simulink model "Arduino_PID_Interface2015b"  (R2015b)
settings: Solver=VariableStepAuto  SolverMode=SingleTasking  StartTime=0.0  StopTime=inf  RelTol=1e-3
undefined symbols (not defined in the file or in its folder): LF, serial
libraries: instrumentlib x3
settings Model: Creator=VM  LastModifiedBy=rap.kuttruf.17
settings DataIOCC: LimitDataPoints=off  ReturnWorkspaceOutputs=on
settings DebuggingCC: AllowSymbolicDim=on  SFUnexpectedBacktrackingDiag=error  SFNoUnconditionalDefaultTransitionDiag=error
settings ModelReferenceCC: PropagateSignalLabelsOutOfModel=on
settings SFSimCC: SimUseLocalCustomCode=on
settings RTWCC: RTWUseLocalCustomCode=on
settings GRTTargetCC: TargetLangStandard=C99 (ISO)
settings ConfigComp: CovMetricSettings=dwe  CovHtmlReporting=off  CovSaveCumulativeToWorkspaceVar=off  CovSaveSingleToWorkspaceVar=off  CovModelRefEnable=Off  CovExternalEMLEnable=on

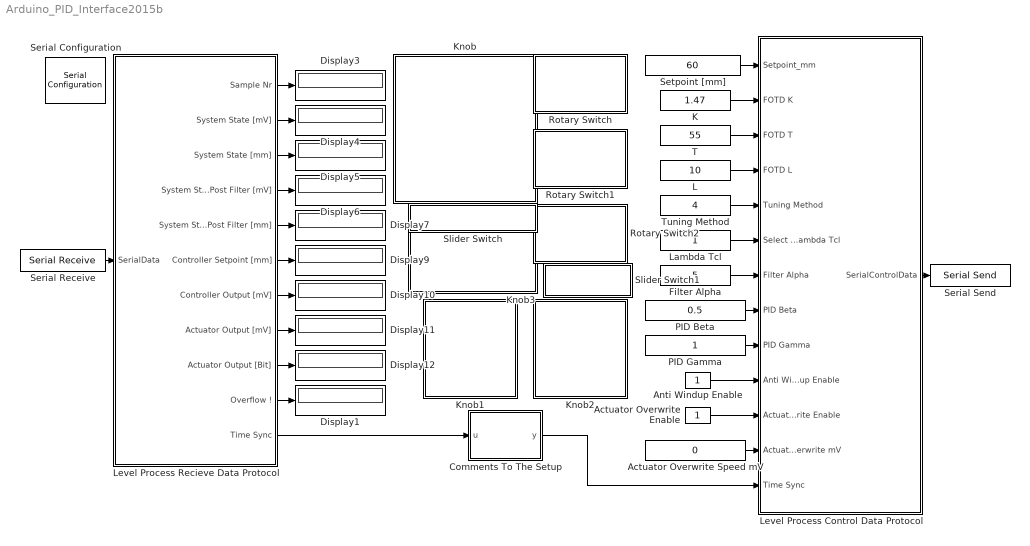
== system Arduino_PID_Interface2015b ==
  Actuator Overwrite Enable : Constant  OutDataTypeStr=uint8
  Actuator Overwrite Speed mV : Constant  Value=0  OutDataTypeStr=double
  Anti Windup Enable : Constant  OutDataTypeStr=uint8
  Comments To The Setup : MATLAB Function  TreatAsAtomicUnit=on
  Display{1,3..7,9..12} (10 alike) : Display
  Filter Alpha : Constant  Value=5
  K : Constant  Value=1.47
  Knob : Subsystem  DialogController=hmiCreateDDGDialog  IsWebBlock=on  mask(MWDashboardBlock){webBlockId=6f032d83-7110-46a9-9e70-2962474ee83c, webBlockType=continuousknob, ShowInLibBrowser=on, ShowInitialText=on, HMISrcModelName=Arduino_PID_Interface2015b}
      mask prompts: webBlockId "WebBlock Id"; webBlockType "WebBlock Type"; HMISrcModelName "Source Model"
      mask help: Set a value to tune parameters or variables.
      mask Help: helpview([docroot '/mapfiles/simulink.map'], 'hmi_knob')
      mask Display:
      | if strcmp(get_param(bdroot(gcb),'BlockDiagramType'),'library')
      |  image([(matlabroot) '/toolbox/simulink/hmi/icons/ContinuousKnob.png'])
      | end
  Knob1 : Subsystem  DialogController=hmiCreateDDGDialog  IsWebBlock=on  mask(MWDashboardBlock){webBlockId=2d92fb6d-6817-4e61-8a75-49afcc5cee09, webBlockType=continuousknob, ShowInLibBrowser=on, ShowInitialText=on, HMISrcModelName=Arduino_PID_Interface2015b}
      mask prompts: webBlockId "WebBlock Id"; webBlockType "WebBlock Type"; HMISrcModelName "Source Model"
      mask help: Set a value to tune parameters or variables.
      mask Help: helpview([docroot '/mapfiles/simulink.map'], 'hmi_knob')
      mask Display:
      | if strcmp(get_param(bdroot(gcb),'BlockDiagramType'),'library')
      |  image([(matlabroot) '/toolbox/simulink/hmi/icons/ContinuousKnob.png'])
      | end
  Knob2 : Subsystem  DialogController=hmiCreateDDGDialog  IsWebBlock=on  mask(MWDashboardBlock){webBlockId=b3bbeefb-f65b-4d0a-99f2-2d47ca17d880, webBlockType=continuousknob, ShowInLibBrowser=on, ShowInitialText=on, HMISrcModelName=Arduino_PID_Interface2015b}
      mask prompts: webBlockId "WebBlock Id"; webBlockType "WebBlock Type"; HMISrcModelName "Source Model"
      mask help: Set a value to tune parameters or variables.
      mask Help: helpview([docroot '/mapfiles/simulink.map'], 'hmi_knob')
      mask Display:
      | if strcmp(get_param(bdroot(gcb),'BlockDiagramType'),'library')
      |  image([(matlabroot) '/toolbox/simulink/hmi/icons/ContinuousKnob.png'])
      | end
  Knob3 : Subsystem  DialogController=hmiCreateDDGDialog  IsWebBlock=on  mask(MWDashboardBlock){webBlockId=3082382d-e086-4832-b15c-b96756403168, webBlockType=continuousknob, ShowInLibBrowser=on, ShowInitialText=on, HMISrcModelName=Arduino_PID_Interface2015b}
      mask prompts: webBlockId "WebBlock Id"; webBlockType "WebBlock Type"; HMISrcModelName "Source Model"
      mask help: Set a value to tune parameters or variables.
      mask Help: helpview([docroot '/mapfiles/simulink.map'], 'hmi_knob')
      mask Display:
      | if strcmp(get_param(bdroot(gcb),'BlockDiagramType'),'library')
      |  image([(matlabroot) '/toolbox/simulink/hmi/icons/ContinuousKnob.png'])
      | end
  L : Constant  Value=10
  Lambda Tcl : Constant
  Level Process Control Data Protocol : Subsystem
  Level Process Recieve Data Protocol : Subsystem
  PID Beta : Constant  Value=0.5
  PID Gamma : Constant
  Rotary Switch : Subsystem  DialogController=hmiCreateDDGDialog  IsWebBlock=on  mask(MWDashboardBlock){webBlockId=54f21b2c-51f9-4bca-8c45-8dfda734ad71, webBlockType=discreteknob, ShowInLibBrowser=on, ShowInitialText=on, HMISrcModelName=Arduino_PID_Interface2015b}
      mask prompts: webBlockId "WebBlock Id"; webBlockType "WebBlock Type"; HMISrcModelName "Source Model"
      mask help: Set value to tune parameters or variables.
      mask Help: helpview([docroot '/mapfiles/simulink.map'], 'hmi_rotary_switch')
      mask Display:
      | if strcmp(get_param(bdroot(gcb),'BlockDiagramType'),'library')
      |  image([(matlabroot) '/toolbox/simulink/hmi/icons/DiscreteKnob.png'])
      | end
  Rotary Switch1 : Subsystem  DialogController=hmiCreateDDGDialog  IsWebBlock=on  mask(MWDashboardBlock){webBlockId=c8a1b7f9-55eb-45f6-8afb-eb5ab7323296, webBlockType=discreteknob, ShowInLibBrowser=on, ShowInitialText=on, HMISrcModelName=Arduino_PID_Interface2015b}
      mask prompts: webBlockId "WebBlock Id"; webBlockType "WebBlock Type"; HMISrcModelName "Source Model"
      mask help: Set value to tune parameters or variables.
      mask Help: helpview([docroot '/mapfiles/simulink.map'], 'hmi_rotary_switch')
      mask Display:
      | if strcmp(get_param(bdroot(gcb),'BlockDiagramType'),'library')
      |  image([(matlabroot) '/toolbox/simulink/hmi/icons/DiscreteKnob.png'])
      | end
  Rotary Switch2 : Subsystem  DialogController=hmiCreateDDGDialog  IsWebBlock=on  mask(MWDashboardBlock){webBlockId=0e63494c-69fc-4820-84ef-30df04359523, webBlockType=discreteknob, ShowInLibBrowser=on, ShowInitialText=on, HMISrcModelName=Arduino_PID_Interface2015b}
      mask prompts: webBlockId "WebBlock Id"; webBlockType "WebBlock Type"; HMISrcModelName "Source Model"
      mask help: Set value to tune parameters or variables.
      mask Help: helpview([docroot '/mapfiles/simulink.map'], 'hmi_rotary_switch')
      mask Display:
      | if strcmp(get_param(bdroot(gcb),'BlockDiagramType'),'library')
      |  image([(matlabroot) '/toolbox/simulink/hmi/icons/DiscreteKnob.png'])
      | end
  Serial Configuration : instrumentlib/Serial Configuration  Priority=-200000  ComPortMenu=<Please select a port...>  ComPort=COM5  ObjConstructor=serial('COM5');  BaudRate=115200  DataBits=8  Parity=none  StopBits=1  FlowControl=none  Timeout=10  ByteOrder=LittleEndian
  Serial Receive : instrumentlib/Serial Receive  ComPortMenu=<Please select a port...>  ComPort=COM5  ObjConstructor=serial('COM5');  Header=<D>  Terminator=LF ('\n')  DataSize="[1  32]"  DataType=uint8  EnableBlockingMode=on  ActionDataUnavailable=Output last received value  CustomValue=0  SampleTime=0.001
  Serial Send : instrumentlib/Serial Send  ComPortMenu=<Please select a port...>  ComPort=COM5  ObjConstructor=serial('COM5');  Header=<C>  Terminator=LF ('\n')  EnableBlockingMode=on
  Setpoint [mm] : Constant  Value=60  OutDataTypeStr=uint16
  Slider Switch : Subsystem  DialogController=hmiCreateDDGDialog  IsWebBlock=on  mask(MWDashboardBlock){webBlockId=4b07397e-e0fe-4bf8-b10b-d486fcba6875, webBlockType=sliderswitch, ShowInLibBrowser=on, ShowInitialText=on, HMISrcModelName=Arduino_PID_Interface2015b}
      mask prompts: webBlockId "WebBlock Id"; webBlockType "WebBlock Type"; HMISrcModelName "Source Model"
      mask help: Set on/off value to tune parameters or variables.
      mask Help: helpview([docroot '/mapfiles/simulink.map'], 'hmi_switch')
      mask Display:
      | if strcmp(get_param(bdroot(gcb),'BlockDiagramType'),'library')
      |  image([(matlabroot) '/toolbox/simulink/hmi/icons/SliderSwitch.png'])
      | end
  Slider Switch1 : Subsystem  DialogController=hmiCreateDDGDialog  IsWebBlock=on  mask(MWDashboardBlock){webBlockId=f5a7a057-55eb-455d-becd-9f4f82eab9b0, webBlockType=sliderswitch, ShowInLibBrowser=on, ShowInitialText=on, HMISrcModelName=Arduino_PID_Interface2015b}
      mask prompts: webBlockId "WebBlock Id"; webBlockType "WebBlock Type"; HMISrcModelName "Source Model"
      mask help: Set on/off value to tune parameters or variables.
      mask Help: helpview([docroot '/mapfiles/simulink.map'], 'hmi_switch')
      mask Display:
      | if strcmp(get_param(bdroot(gcb),'BlockDiagramType'),'library')
      |  image([(matlabroot) '/toolbox/simulink/hmi/icons/SliderSwitch.png'])
      | end
  T : Constant  Value=55
  Tuning Method : Constant  Value=4
  wires:
  Serial Receive/1 -> Level Process Recieve Data Protocol/1(SerialData)
  Setpoint [mm]/1 -> Level Process Control Data Protocol/1(Setpoint_mm)
  Level Process Recieve Data Protocol/1(Sample Nr) -> Display3/1
  Level Process Recieve Data Protocol/2(System State [mV]) -> Display4/1
  Level Process Recieve Data Protocol/3(System State [mm]) -> Display5/1
  Level Process Recieve Data Protocol/4(System State Post Filter [mV]) -> Display6/1
  Level Process Recieve Data Protocol/5(System State Post Filter [mm]) -> Display7/1
  Level Process Recieve Data Protocol/6(Controller Setpoint [mm]) -> Display9/1
  Level Process Recieve Data Protocol/7(Controller Output [mV]) -> Display10/1
  Level Process Recieve Data Protocol/8(Actuator Output [mV]) -> Display11/1
  Level Process Recieve Data Protocol/9(Actuator Output [Bit]) -> Display12/1
  Tuning Method/1 -> Level Process Control Data Protocol/5(Tuning Method)
  Filter Alpha/1 -> Level Process Control Data Protocol/7(Filter Alpha)
  Level Process Control Data Protocol/1(SerialControlData) -> Serial Send/1
  K/1 -> Level Process Control Data Protocol/2(FOTD K)
  PID Beta/1 -> Level Process Control Data Protocol/8(PID Beta)
  PID Gamma/1 -> Level Process Control Data Protocol/9(PID Gamma)
  T/1 -> Level Process Control Data Protocol/3(FOTD T)
  L/1 -> Level Process Control Data Protocol/4(FOTD L)
  Lambda Tcl/1 -> Level Process Control Data Protocol/6(Select Lambda Tcl)
  Level Process Recieve Data Protocol/11(Time Sync) -> Comments To The Setup/1(u)
  Comments To The Setup/1(y) -> Level Process Control Data Protocol/13(Time Sync)
  Level Process Recieve Data Protocol/10(Overflow !) -> Display1/1
  Actuator Overwrite Speed mV/1 -> Level Process Control Data Protocol/12(Actuator Speed Overwrite mV)
  Actuator Overwrite Enable/1 -> Level Process Control Data Protocol/11(Actuator Overwrite Enable)
  Anti Windup Enable/1 -> Level Process Control Data Protocol/10(Anti Windup Enable)

== system Arduino_PID_Interface2015b/Knob ==

== system Arduino_PID_Interface2015b/Knob1 ==

== system Arduino_PID_Interface2015b/Knob2 ==

== system Arduino_PID_Interface2015b/Knob3 ==

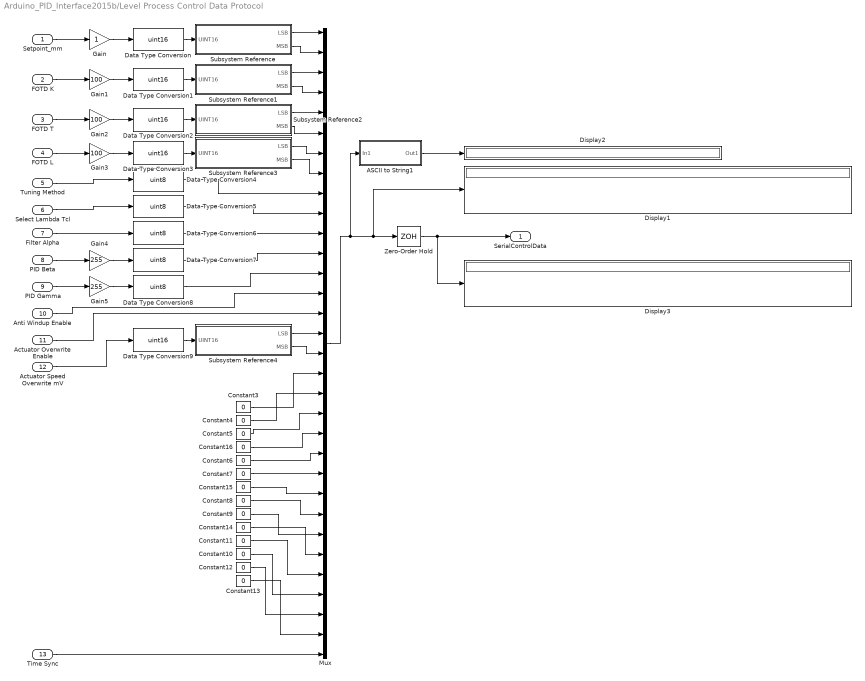
== system Arduino_PID_Interface2015b/Level Process Control Data Protocol ==
  Setpoint_mm : Inport
  FOTD K : Inport  Port=2
  FOTD T : Inport  Port=3
  FOTD L : Inport  Port=4
  Tuning Method : Inport  Port=5
  Select Lambda Tcl : Inport  Port=6
  Filter Alpha : Inport  Port=7
  PID Beta : Inport  Port=8
  PID Gamma : Inport  Port=9
  Anti Windup Enable : Inport  Port=10
  Actuator Overwrite Enable : Inport  Port=11
  Actuator Speed Overwrite mV : Inport  Port=12
  Time Sync : Inport  Port=13
  ASCII to String1 : Subsystem  Description=Replaced Block  mask(Replaced Block){}
      mask help: This block has been replaced with an empty subsystem because it used functionality that is unavailable in Simulink R2015b.
      mask Display: fprintf('Replaced: %s\n','ASCIIToString')
  Constant{3..16} (14 alike) : Constant  Value=0  OutDataTypeStr=uint8
  Data Type Conversion{,1..3,9} (5 alike) : DataTypeConversion  OutDataTypeStr=uint16
  Data Type Conversion{4..8} (5 alike) : DataTypeConversion  OutDataTypeStr=uint8
  Display1 : Display
      settings: Decimation=32
  Display2 : Display
  Display3 : Display
      settings: Decimation=32
  Gain : Gain
  Gain1 : Gain  Gain=100
  Gain2 : Gain  Gain=100
  Gain3 : Gain  Gain=100
  Gain4 : Gain  Gain=255
  Gain5 : Gain  Gain=255
  Mux : Mux  Inputs=32
  Subsystem Reference : Subsystem
  Subsystem Reference1 : Subsystem
  Subsystem Reference2 : Subsystem
  Subsystem Reference3 : Subsystem
  Subsystem Reference4 : Subsystem
  Zero-Order Hold : ZeroOrderHold  SampleTime=0.005
  SerialControlData : Outport
  wires:
  Subsystem Reference/1(LSB) -> Mux/1
  Subsystem Reference/2(MSB) -> Mux/2
  Data Type Conversion/1 -> Subsystem Reference/1(UINT16)
  Gain/1 -> Data Type Conversion/1
  Setpoint_mm/1 -> Gain/1
  Gain1/1 -> Data Type Conversion1/1
  Data Type Conversion1/1 -> Subsystem Reference1/1(UINT16)
  Subsystem Reference1/1(LSB) -> Mux/3
  Subsystem Reference1/2(MSB) -> Mux/4
  Gain2/1 -> Data Type Conversion2/1
  Data Type Conversion2/1 -> Subsystem Reference2/1(UINT16)
  Subsystem Reference2/1(LSB) -> Mux/5
  Subsystem Reference2/2(MSB) -> Mux/6
  Gain3/1 -> Data Type Conversion3/1
  Data Type Conversion3/1 -> Subsystem Reference3/1(UINT16)
  Subsystem Reference3/1(LSB) -> Mux/7
  Subsystem Reference3/2(MSB) -> Mux/8
  FOTD K/1 -> Gain1/1
  FOTD T/1 -> Gain2/1
  FOTD L/1 -> Gain3/1
  Tuning Method/1 -> Data Type Conversion4/1
  Data Type Conversion4/1 -> Mux/9
  Select Lambda Tcl/1 -> Data Type Conversion5/1
  Filter Alpha/1 -> Data Type Conversion6/1
  Data Type Conversion5/1 -> Mux/10
  Data Type Conversion6/1 -> Mux/11
  Data Type Conversion7/1 -> Mux/12
  Data Type Conversion8/1 -> Mux/13
  ASCII to String1/1(Out1) -> Display2/1
  Mux/1 -> ASCII to String1/1(In1), Zero-Order Hold/1, Display1/1
  PID Beta/1 -> Gain4/1
  Gain4/1 -> Data Type Conversion7/1
  PID Gamma/1 -> Gain5/1
  Gain5/1 -> Data Type Conversion8/1
  Time Sync/1 -> Mux/32
  Constant3/1 -> Mux/18
  Constant4/1 -> Mux/19
  Constant5/1 -> Mux/20
  Constant6/1 -> Mux/22
  Constant7/1 -> Mux/23
  Constant8/1 -> Mux/25
  Constant9/1 -> Mux/26
  Constant10/1 -> Mux/29
  Constant11/1 -> Mux/28
  Constant12/1 -> Mux/30
  Constant13/1 -> Mux/31
  Constant15/1 -> Mux/24
  Constant16/1 -> Mux/21
  Constant14/1 -> Mux/27
  Data Type Conversion9/1 -> Subsystem Reference4/1(UINT16)
  Actuator Speed Overwrite mV/1 -> Data Type Conversion9/1
  Zero-Order Hold/1 -> Display3/1, SerialControlData/1
  Subsystem Reference4/1(LSB) -> Mux/16
  Subsystem Reference4/2(MSB) -> Mux/17
  Actuator Overwrite Enable/1 -> Mux/15
  Anti Windup Enable/1 -> Mux/14

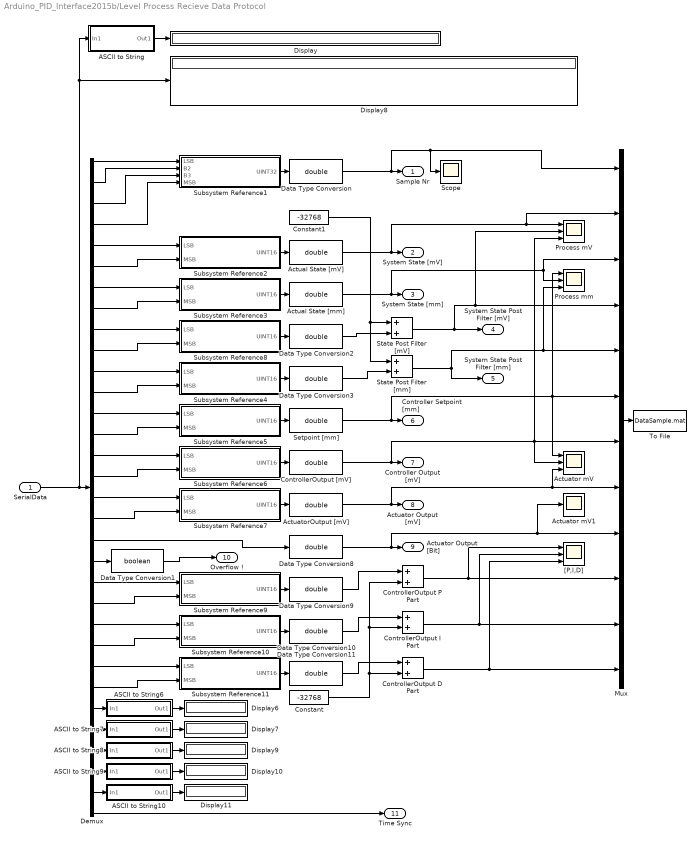
== system Arduino_PID_Interface2015b/Level Process Recieve Data Protocol ==
  SerialData : Inport
  " Actual State [mV]" : DataTypeConversion  OutDataTypeStr=double
  " Actual State [mm]" : DataTypeConversion  OutDataTypeStr=double
  ASCII to String : Subsystem  Description=Replaced Block  mask(Replaced Block){}
      mask help: This block has been replaced with an empty subsystem because it used functionality that is unavailable in Simulink R2015b.
      mask Display: fprintf('Replaced: %s\n','ASCIIToString')
  ASCII to String10 : Subsystem  Description=Replaced Block  mask(Replaced Block){}
      mask help: This block has been replaced with an empty subsystem because it used functionality that is unavailable in Simulink R2015b.
      mask Display: fprintf('Replaced: %s\n','ASCIIToString')
  ASCII to String6 : Subsystem  Description=Replaced Block  mask(Replaced Block){}
      mask help: This block has been replaced with an empty subsystem because it used functionality that is unavailable in Simulink R2015b.
      mask Display: fprintf('Replaced: %s\n','ASCIIToString')
  ASCII to String7 : Subsystem  Description=Replaced Block  mask(Replaced Block){}
      mask help: This block has been replaced with an empty subsystem because it used functionality that is unavailable in Simulink R2015b.
      mask Display: fprintf('Replaced: %s\n','ASCIIToString')
  ASCII to String8 : Subsystem  Description=Replaced Block  mask(Replaced Block){}
      mask help: This block has been replaced with an empty subsystem because it used functionality that is unavailable in Simulink R2015b.
      mask Display: fprintf('Replaced: %s\n','ASCIIToString')
  ASCII to String9 : Subsystem  Description=Replaced Block  mask(Replaced Block){}
      mask help: This block has been replaced with an empty subsystem because it used functionality that is unavailable in Simulink R2015b.
      mask Display: fprintf('Replaced: %s\n','ASCIIToString')
  Actuator mV : Scope  NumInputPorts=3
  Actuator mV1 : Scope
  ActuatorOutput [mV] : DataTypeConversion  OutDataTypeStr=double
  Constant : Constant  Value=-32768
  Constant1 : Constant  Value=-32768
  ControllerOutput D Part : Sum
  ControllerOutput I Part : Sum
  ControllerOutput P Part : Sum
  ControllerOutput [mV] : DataTypeConversion  OutDataTypeStr=double
  Data Type Conversion{,2..3,8..11} (7 alike) : DataTypeConversion  OutDataTypeStr=double
  Data Type Conversion1 : DataTypeConversion  OutDataTypeStr=boolean
  Demux : Demux  Outputs=32
  Display{,6..11} (7 alike) : Display
      Display8 settings: Decimation=32
  Mux : Mux  Inputs=12
  Process mV : Scope  NumInputPorts=3
  Process mm : Scope  NumInputPorts=3
  Scope : Scope
  Setpoint [mm] : DataTypeConversion  OutDataTypeStr=double
  State Post Filter [mV] : Sum
  State Post Filter [mm] : Sum
  Subsystem Reference1 : Subsystem
  Subsystem Reference10 : Subsystem
  Subsystem Reference11 : Subsystem
  Subsystem Reference2 : Subsystem
  Subsystem Reference3 : Subsystem
  Subsystem Reference4 : Subsystem
  Subsystem Reference5 : Subsystem
  Subsystem Reference6 : Subsystem
  Subsystem Reference7 : Subsystem
  Subsystem Reference8 : Subsystem
  Subsystem Reference9 : Subsystem
  To File : ToFile  Filename=DataSample.mat  MatrixName=DataSample  SaveFormat=Timeseries
  "[P,I,D]" : Scope  NumInputPorts=3
  Sample Nr : Outport
  System State [mV] : Outport  Port=2
  System State [mm] : Outport  Port=3
  System State Post Filter [mV] : Outport  Port=4
  System State Post Filter [mm] : Outport  Port=5
  Controller Setpoint [mm] : Outport  Port=6
  Controller Output [mV] : Outport  Port=7
  Actuator Output [mV] : Outport  Port=8
  Actuator Output [Bit] : Outport  Port=9
  Overflow ! : Outport  Port=10  OutDataTypeStr=boolean
  Time Sync : Outport  Port=11
  wires:
  SerialData/1 -> ASCII to String/1(In1), Display8/1, Demux/1
  Demux/2 -> Subsystem Reference1/2(B2)
  Demux/1 -> Subsystem Reference1/1(LSB)
  Demux/3 -> Subsystem Reference1/3(B3)
  Demux/4 -> Subsystem Reference1/4(MSB)
  Demux/17 -> Subsystem Reference7/1(LSB)
  Demux/18 -> Subsystem Reference7/2(MSB)
  Subsystem Reference1/1(UINT32) -> Data Type Conversion/1
  Subsystem Reference7/1(UINT16) -> ActuatorOutput [mV]/1
  Demux/19 -> Data Type Conversion8/1
  Data Type Conversion/1 -> Scope/1, Mux/1, Sample Nr/1
  " Actual State [mV]"/1 -> Mux/2, Process mV/1, System State [mV]/1
  " Actual State [mm]"/1 -> Process mm/2, Mux/3, System State [mm]/1
  Setpoint [mm]/1 -> Process mm/1, Mux/6, Actuator mV/1, Controller Setpoint [mm]/1
  ControllerOutput [mV]/1 -> Actuator mV/2, Mux/7, Process mV/3, Controller Output [mV]/1
  ActuatorOutput [mV]/1 -> Actuator mV/3, Mux/8, Actuator Output [mV]/1
  Data Type Conversion8/1 -> Actuator mV1/1, Mux/9, Actuator Output [Bit]/1
  ASCII to String/1(Out1) -> Display/1
  Mux/1 -> To File/1
  Demux/32 -> Time Sync/1
  ASCII to String6/1(Out1) -> Display6/1
  Demux/27 -> ASCII to String6/1(In1)
  ASCII to String7/1(Out1) -> Display7/1
  Demux/28 -> ASCII to String7/1(In1)
  ASCII to String8/1(Out1) -> Display9/1
  Demux/29 -> ASCII to String8/1(In1)
  ASCII to String9/1(Out1) -> Display10/1
  Demux/30 -> ASCII to String9/1(In1)
  ASCII to String10/1(Out1) -> Display11/1
  Demux/31 -> ASCII to String10/1(In1)
  Subsystem Reference2/1(UINT16) -> " Actual State [mV]"/1
  Subsystem Reference3/1(UINT16) -> " Actual State [mm]"/1
  Subsystem Reference5/1(UINT16) -> Setpoint [mm]/1
  Subsystem Reference6/1(UINT16) -> ControllerOutput [mV]/1
  Demux/5 -> Subsystem Reference2/1(LSB)
  Demux/6 -> Subsystem Reference2/2(MSB)
  Demux/7 -> Subsystem Reference3/1(LSB)
  Demux/9 -> Subsystem Reference8/1(LSB)
  Demux/11 -> Subsystem Reference4/1(LSB)
  Demux/13 -> Subsystem Reference5/1(LSB)
  Demux/15 -> Subsystem Reference6/1(LSB)
  Demux/16 -> Subsystem Reference6/2(MSB)
  Demux/14 -> Subsystem Reference5/2(MSB)
  Demux/12 -> Subsystem Reference4/2(MSB)
  Demux/10 -> Subsystem Reference8/2(MSB)
  Demux/8 -> Subsystem Reference3/2(MSB)
  Demux/21 -> Subsystem Reference9/1(LSB)
  Demux/22 -> Subsystem Reference9/2(MSB)
  Demux/23 -> Subsystem Reference10/1(LSB)
  Demux/24 -> Subsystem Reference10/2(MSB)
  Demux/25 -> Subsystem Reference11/1(LSB)
  Demux/26 -> Subsystem Reference11/2(MSB)
  Subsystem Reference9/1(UINT16) -> Data Type Conversion9/1
  Subsystem Reference10/1(UINT16) -> Data Type Conversion10/1
  Subsystem Reference11/1(UINT16) -> Data Type Conversion11/1
  Data Type Conversion9/1 -> ControllerOutput P Part/1
  Data Type Conversion11/1 -> ControllerOutput D Part/1
  Data Type Conversion10/1 -> ControllerOutput I Part/1
  Constant/1 -> ControllerOutput D Part/2, ControllerOutput I Part/2, ControllerOutput P Part/2
  ControllerOutput P Part/1 -> "[P,I,D]"/1, Mux/10
  ControllerOutput I Part/1 -> "[P,I,D]"/2, Mux/11
  ControllerOutput D Part/1 -> Mux/12, "[P,I,D]"/3
  Data Type Conversion1/1 -> Overflow !/1
  Demux/20 -> Data Type Conversion1/1
  State Post Filter [mV]/1 -> System State Post Filter [mV]/1, Mux/4, Process mV/2
  Constant1/1 -> State Post Filter [mV]/1, State Post Filter [mm]/1
  Subsystem Reference8/1(UINT16) -> Data Type Conversion2/1
  Data Type Conversion2/1 -> State Post Filter [mV]/2
  Subsystem Reference4/1(UINT16) -> Data Type Conversion3/1
  Data Type Conversion3/1 -> State Post Filter [mm]/2
  State Post Filter [mm]/1 -> Mux/5, Process mm/3, System State Post Filter [mm]/1

== system Arduino_PID_Interface2015b/Rotary Switch ==

== system Arduino_PID_Interface2015b/Rotary Switch1 ==

== system Arduino_PID_Interface2015b/Rotary Switch2 ==

== system Arduino_PID_Interface2015b/Slider Switch ==

== system Arduino_PID_Interface2015b/Slider Switch1 ==

== system Arduino_PID_Interface2015b/Level Process Control Data Protocol/ASCII to String1 ==
  In1 : Inport
  Ground1 : Ground
  Terminator1 : Terminator
  Out1 : Outport
  wires:
  Ground1/1 -> Out1/1
  In1/1 -> Terminator1/1

== system Arduino_PID_Interface2015b/Level Process Control Data Protocol/Subsystem Reference ==
  UINT16 : Inport  OutDataTypeStr=uint16
  Data Type Conversion : DataTypeConversion  OutDataTypeStr=uint8
  Data Type Conversion1 : DataTypeConversion  OutDataTypeStr=uint8
  Data Type Conversion2 : DataTypeConversion  OutDataTypeStr=uint8  ConvertRealWorld=Stored Integer (SI)
  Display{,1..3} (4 alike) : Display
  Shift Arithmetic : ArithShift  BitShiftNumber=8  BitShiftDirection=Right
  LSB : Outport
  MSB : Outport  Port=2
  wires:
  Data Type Conversion2/1 -> Data Type Conversion/1, Display/1
  Data Type Conversion/1 -> LSB/1, Display2/1
  Data Type Conversion1/1 -> MSB/1, Display3/1
  Shift Arithmetic/1 -> Data Type Conversion1/1, Display1/1
  UINT16/1 -> Shift Arithmetic/1, Data Type Conversion2/1

== system Arduino_PID_Interface2015b/Level Process Control Data Protocol/Subsystem Reference1 ==
  UINT16 : Inport  OutDataTypeStr=uint16
  Data Type Conversion : DataTypeConversion  OutDataTypeStr=uint8
  Data Type Conversion1 : DataTypeConversion  OutDataTypeStr=uint8
  Data Type Conversion2 : DataTypeConversion  OutDataTypeStr=uint8  ConvertRealWorld=Stored Integer (SI)
  Display{,1..3} (4 alike) : Display
  Shift Arithmetic : ArithShift  BitShiftNumber=8  BitShiftDirection=Right
  LSB : Outport
  MSB : Outport  Port=2
  wires:
  Data Type Conversion2/1 -> Data Type Conversion/1, Display/1
  Data Type Conversion/1 -> LSB/1, Display2/1
  Data Type Conversion1/1 -> MSB/1, Display3/1
  Shift Arithmetic/1 -> Data Type Conversion1/1, Display1/1
  UINT16/1 -> Shift Arithmetic/1, Data Type Conversion2/1

== system Arduino_PID_Interface2015b/Level Process Control Data Protocol/Subsystem Reference2 ==
  UINT16 : Inport  OutDataTypeStr=uint16
  Data Type Conversion : DataTypeConversion  OutDataTypeStr=uint8
  Data Type Conversion1 : DataTypeConversion  OutDataTypeStr=uint8
  Data Type Conversion2 : DataTypeConversion  OutDataTypeStr=uint8  ConvertRealWorld=Stored Integer (SI)
  Display{,1..3} (4 alike) : Display
  Shift Arithmetic : ArithShift  BitShiftNumber=8  BitShiftDirection=Right
  LSB : Outport
  MSB : Outport  Port=2
  wires:
  Data Type Conversion2/1 -> Data Type Conversion/1, Display/1
  Data Type Conversion/1 -> LSB/1, Display2/1
  Data Type Conversion1/1 -> MSB/1, Display3/1
  Shift Arithmetic/1 -> Data Type Conversion1/1, Display1/1
  UINT16/1 -> Shift Arithmetic/1, Data Type Conversion2/1

== system Arduino_PID_Interface2015b/Level Process Control Data Protocol/Subsystem Reference3 ==
  UINT16 : Inport  OutDataTypeStr=uint16
  Data Type Conversion : DataTypeConversion  OutDataTypeStr=uint8
  Data Type Conversion1 : DataTypeConversion  OutDataTypeStr=uint8
  Data Type Conversion2 : DataTypeConversion  OutDataTypeStr=uint8  ConvertRealWorld=Stored Integer (SI)
  Display{,1..3} (4 alike) : Display
  Shift Arithmetic : ArithShift  BitShiftNumber=8  BitShiftDirection=Right
  LSB : Outport
  MSB : Outport  Port=2
  wires:
  Data Type Conversion2/1 -> Data Type Conversion/1, Display/1
  Data Type Conversion/1 -> LSB/1, Display2/1
  Data Type Conversion1/1 -> MSB/1, Display3/1
  Shift Arithmetic/1 -> Data Type Conversion1/1, Display1/1
  UINT16/1 -> Shift Arithmetic/1, Data Type Conversion2/1

== system Arduino_PID_Interface2015b/Level Process Control Data Protocol/Subsystem Reference4 ==
  UINT16 : Inport  OutDataTypeStr=uint16
  Data Type Conversion : DataTypeConversion  OutDataTypeStr=uint8
  Data Type Conversion1 : DataTypeConversion  OutDataTypeStr=uint8
  Data Type Conversion2 : DataTypeConversion  OutDataTypeStr=uint8  ConvertRealWorld=Stored Integer (SI)
  Display{,1..3} (4 alike) : Display
  Shift Arithmetic : ArithShift  BitShiftNumber=8  BitShiftDirection=Right
  LSB : Outport
  MSB : Outport  Port=2
  wires:
  Data Type Conversion2/1 -> Data Type Conversion/1, Display/1
  Data Type Conversion/1 -> LSB/1, Display2/1
  Data Type Conversion1/1 -> MSB/1, Display3/1
  Shift Arithmetic/1 -> Data Type Conversion1/1, Display1/1
  UINT16/1 -> Shift Arithmetic/1, Data Type Conversion2/1

== system Arduino_PID_Interface2015b/Level Process Recieve Data Protocol/ASCII to String ==
  In1 : Inport
  Ground1 : Ground
  Terminator1 : Terminator
  Out1 : Outport
  wires:
  Ground1/1 -> Out1/1
  In1/1 -> Terminator1/1

== system Arduino_PID_Interface2015b/Level Process Recieve Data Protocol/ASCII to String10 ==
  In1 : Inport
  Ground1 : Ground
  Terminator1 : Terminator
  Out1 : Outport
  wires:
  Ground1/1 -> Out1/1
  In1/1 -> Terminator1/1

== system Arduino_PID_Interface2015b/Level Process Recieve Data Protocol/ASCII to String6 ==
  In1 : Inport
  Ground1 : Ground
  Terminator1 : Terminator
  Out1 : Outport
  wires:
  Ground1/1 -> Out1/1
  In1/1 -> Terminator1/1

== system Arduino_PID_Interface2015b/Level Process Recieve Data Protocol/ASCII to String7 ==
  In1 : Inport
  Ground1 : Ground
  Terminator1 : Terminator
  Out1 : Outport
  wires:
  Ground1/1 -> Out1/1
  In1/1 -> Terminator1/1

== system Arduino_PID_Interface2015b/Level Process Recieve Data Protocol/ASCII to String8 ==
  In1 : Inport
  Ground1 : Ground
  Terminator1 : Terminator
  Out1 : Outport
  wires:
  Ground1/1 -> Out1/1
  In1/1 -> Terminator1/1

== system Arduino_PID_Interface2015b/Level Process Recieve Data Protocol/ASCII to String9 ==
  In1 : Inport
  Ground1 : Ground
  Terminator1 : Terminator
  Out1 : Outport
  wires:
  Ground1/1 -> Out1/1
  In1/1 -> Terminator1/1

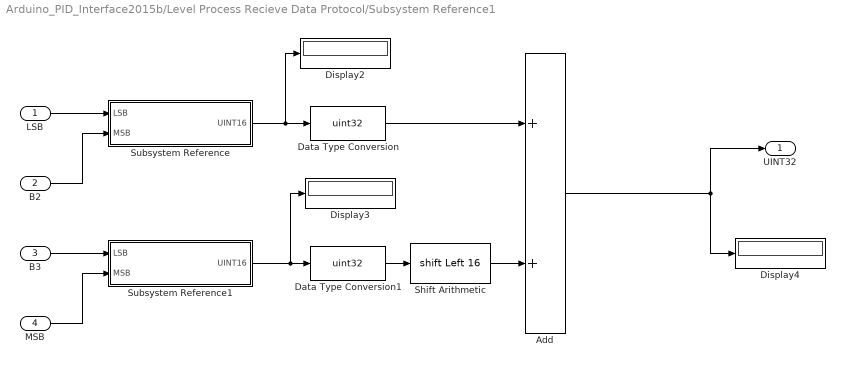
== system Arduino_PID_Interface2015b/Level Process Recieve Data Protocol/Subsystem Reference1 ==
  LSB : Inport  OutDataTypeStr=uint8
  B2 : Inport  Port=2  OutDataTypeStr=uint8
  B3 : Inport  Port=3  OutDataTypeStr=uint8
  MSB : Inport  Port=4  OutDataTypeStr=uint8
  Add : Sum
  Data Type Conversion : DataTypeConversion  OutDataTypeStr=uint32
  Data Type Conversion1 : DataTypeConversion  OutDataTypeStr=uint32
  Display2 : Display
  Display3 : Display
  Display4 : Display
  Shift Arithmetic : ArithShift  BitShiftNumber=16  BitShiftDirection=Left
  Subsystem Reference : Subsystem
  Subsystem Reference1 : Subsystem
  UINT32 : Outport  OutDataTypeStr=uint32  LockScale=on
  wires:
  Shift Arithmetic/1 -> Add/2
  Data Type Conversion/1 -> Add/1
  Add/1 -> Display4/1, UINT32/1
  Data Type Conversion1/1 -> Shift Arithmetic/1
  Subsystem Reference1/1(UINT16) -> Display3/1, Data Type Conversion1/1
  Subsystem Reference/1(UINT16) -> Display2/1, Data Type Conversion/1
  LSB/1 -> Subsystem Reference/1(LSB)
  B2/1 -> Subsystem Reference/2(MSB)
  B3/1 -> Subsystem Reference1/1(LSB)
  MSB/1 -> Subsystem Reference1/2(MSB)

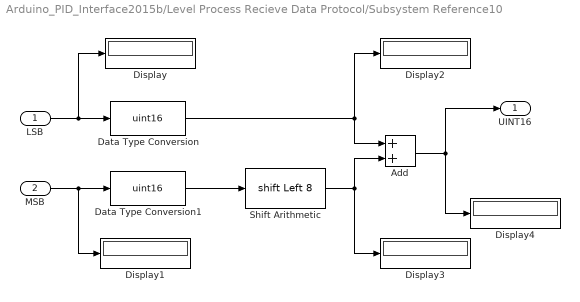
== system Arduino_PID_Interface2015b/Level Process Recieve Data Protocol/Subsystem Reference10 ==
  LSB : Inport  OutDataTypeStr=uint8
  MSB : Inport  Port=2  OutDataTypeStr=uint8
  Add : Sum
  Data Type Conversion : DataTypeConversion  OutDataTypeStr=uint16
  Data Type Conversion1 : DataTypeConversion  OutDataTypeStr=uint16
  Display{,1..4} (5 alike) : Display
  Shift Arithmetic : ArithShift  BitShiftNumber=8  BitShiftDirection=Left
  UINT16 : Outport  OutDataTypeStr=uint16  LockScale=on
  wires:
  LSB/1 -> Data Type Conversion/1, Display/1
  Shift Arithmetic/1 -> Add/2, Display3/1
  Data Type Conversion/1 -> Add/1, Display2/1
  Add/1 -> UINT16/1, Display4/1
  MSB/1 -> Data Type Conversion1/1, Display1/1
  Data Type Conversion1/1 -> Shift Arithmetic/1

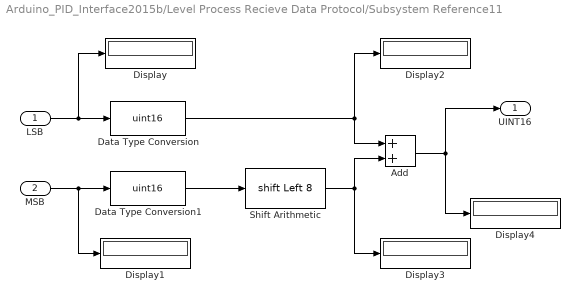
== system Arduino_PID_Interface2015b/Level Process Recieve Data Protocol/Subsystem Reference11 ==
  LSB : Inport  OutDataTypeStr=uint8
  MSB : Inport  Port=2  OutDataTypeStr=uint8
  Add : Sum
  Data Type Conversion : DataTypeConversion  OutDataTypeStr=uint16
  Data Type Conversion1 : DataTypeConversion  OutDataTypeStr=uint16
  Display{,1..4} (5 alike) : Display
  Shift Arithmetic : ArithShift  BitShiftNumber=8  BitShiftDirection=Left
  UINT16 : Outport  OutDataTypeStr=uint16  LockScale=on
  wires:
  LSB/1 -> Data Type Conversion/1, Display/1
  Shift Arithmetic/1 -> Add/2, Display3/1
  Data Type Conversion/1 -> Add/1, Display2/1
  Add/1 -> UINT16/1, Display4/1
  MSB/1 -> Data Type Conversion1/1, Display1/1
  Data Type Conversion1/1 -> Shift Arithmetic/1

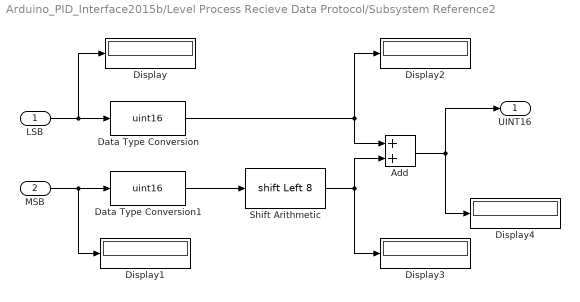
== system Arduino_PID_Interface2015b/Level Process Recieve Data Protocol/Subsystem Reference2 ==
  LSB : Inport  OutDataTypeStr=uint8
  MSB : Inport  Port=2  OutDataTypeStr=uint8
  Add : Sum
  Data Type Conversion : DataTypeConversion  OutDataTypeStr=uint16
  Data Type Conversion1 : DataTypeConversion  OutDataTypeStr=uint16
  Display{,1..4} (5 alike) : Display
  Shift Arithmetic : ArithShift  BitShiftNumber=8  BitShiftDirection=Left
  UINT16 : Outport  OutDataTypeStr=uint16  LockScale=on
  wires:
  LSB/1 -> Data Type Conversion/1, Display/1
  Shift Arithmetic/1 -> Add/2, Display3/1
  Data Type Conversion/1 -> Add/1, Display2/1
  Add/1 -> UINT16/1, Display4/1
  MSB/1 -> Data Type Conversion1/1, Display1/1
  Data Type Conversion1/1 -> Shift Arithmetic/1

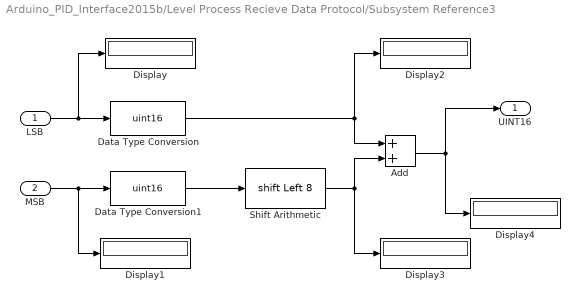
== system Arduino_PID_Interface2015b/Level Process Recieve Data Protocol/Subsystem Reference3 ==
  LSB : Inport  OutDataTypeStr=uint8
  MSB : Inport  Port=2  OutDataTypeStr=uint8
  Add : Sum
  Data Type Conversion : DataTypeConversion  OutDataTypeStr=uint16
  Data Type Conversion1 : DataTypeConversion  OutDataTypeStr=uint16
  Display{,1..4} (5 alike) : Display
  Shift Arithmetic : ArithShift  BitShiftNumber=8  BitShiftDirection=Left
  UINT16 : Outport  OutDataTypeStr=uint16  LockScale=on
  wires:
  LSB/1 -> Data Type Conversion/1, Display/1
  Shift Arithmetic/1 -> Add/2, Display3/1
  Data Type Conversion/1 -> Add/1, Display2/1
  Add/1 -> UINT16/1, Display4/1
  MSB/1 -> Data Type Conversion1/1, Display1/1
  Data Type Conversion1/1 -> Shift Arithmetic/1

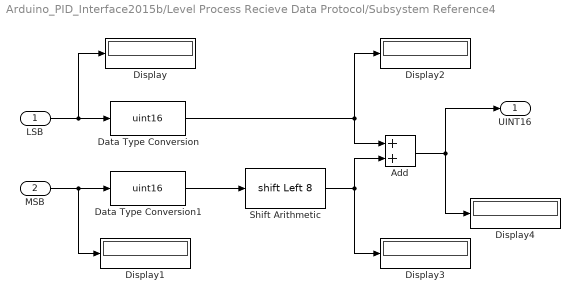
== system Arduino_PID_Interface2015b/Level Process Recieve Data Protocol/Subsystem Reference4 ==
  LSB : Inport  OutDataTypeStr=uint8
  MSB : Inport  Port=2  OutDataTypeStr=uint8
  Add : Sum
  Data Type Conversion : DataTypeConversion  OutDataTypeStr=uint16
  Data Type Conversion1 : DataTypeConversion  OutDataTypeStr=uint16
  Display{,1..4} (5 alike) : Display
  Shift Arithmetic : ArithShift  BitShiftNumber=8  BitShiftDirection=Left
  UINT16 : Outport  OutDataTypeStr=uint16  LockScale=on
  wires:
  LSB/1 -> Data Type Conversion/1, Display/1
  Shift Arithmetic/1 -> Add/2, Display3/1
  Data Type Conversion/1 -> Add/1, Display2/1
  Add/1 -> UINT16/1, Display4/1
  MSB/1 -> Data Type Conversion1/1, Display1/1
  Data Type Conversion1/1 -> Shift Arithmetic/1

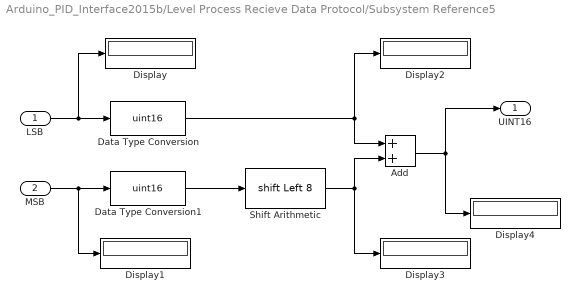
== system Arduino_PID_Interface2015b/Level Process Recieve Data Protocol/Subsystem Reference5 ==
  LSB : Inport  OutDataTypeStr=uint8
  MSB : Inport  Port=2  OutDataTypeStr=uint8
  Add : Sum
  Data Type Conversion : DataTypeConversion  OutDataTypeStr=uint16
  Data Type Conversion1 : DataTypeConversion  OutDataTypeStr=uint16
  Display{,1..4} (5 alike) : Display
  Shift Arithmetic : ArithShift  BitShiftNumber=8  BitShiftDirection=Left
  UINT16 : Outport  OutDataTypeStr=uint16  LockScale=on
  wires:
  LSB/1 -> Data Type Conversion/1, Display/1
  Shift Arithmetic/1 -> Add/2, Display3/1
  Data Type Conversion/1 -> Add/1, Display2/1
  Add/1 -> UINT16/1, Display4/1
  MSB/1 -> Data Type Conversion1/1, Display1/1
  Data Type Conversion1/1 -> Shift Arithmetic/1

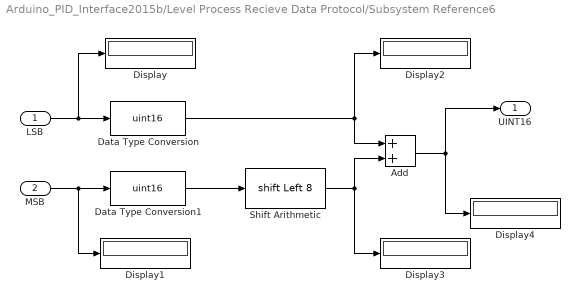
== system Arduino_PID_Interface2015b/Level Process Recieve Data Protocol/Subsystem Reference6 ==
  LSB : Inport  OutDataTypeStr=uint8
  MSB : Inport  Port=2  OutDataTypeStr=uint8
  Add : Sum
  Data Type Conversion : DataTypeConversion  OutDataTypeStr=uint16
  Data Type Conversion1 : DataTypeConversion  OutDataTypeStr=uint16
  Display{,1..4} (5 alike) : Display
  Shift Arithmetic : ArithShift  BitShiftNumber=8  BitShiftDirection=Left
  UINT16 : Outport  OutDataTypeStr=uint16  LockScale=on
  wires:
  LSB/1 -> Data Type Conversion/1, Display/1
  Shift Arithmetic/1 -> Add/2, Display3/1
  Data Type Conversion/1 -> Add/1, Display2/1
  Add/1 -> UINT16/1, Display4/1
  MSB/1 -> Data Type Conversion1/1, Display1/1
  Data Type Conversion1/1 -> Shift Arithmetic/1

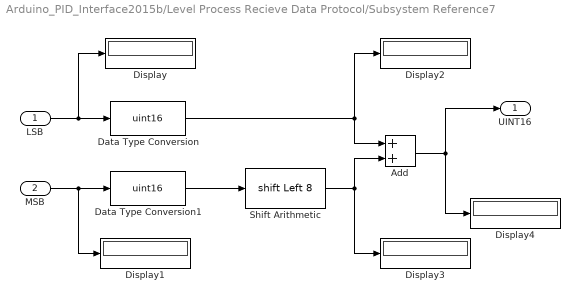
== system Arduino_PID_Interface2015b/Level Process Recieve Data Protocol/Subsystem Reference7 ==
  LSB : Inport  OutDataTypeStr=uint8
  MSB : Inport  Port=2  OutDataTypeStr=uint8
  Add : Sum
  Data Type Conversion : DataTypeConversion  OutDataTypeStr=uint16
  Data Type Conversion1 : DataTypeConversion  OutDataTypeStr=uint16
  Display{,1..4} (5 alike) : Display
  Shift Arithmetic : ArithShift  BitShiftNumber=8  BitShiftDirection=Left
  UINT16 : Outport  OutDataTypeStr=uint16  LockScale=on
  wires:
  LSB/1 -> Data Type Conversion/1, Display/1
  Shift Arithmetic/1 -> Add/2, Display3/1
  Data Type Conversion/1 -> Add/1, Display2/1
  Add/1 -> UINT16/1, Display4/1
  MSB/1 -> Data Type Conversion1/1, Display1/1
  Data Type Conversion1/1 -> Shift Arithmetic/1

== system Arduino_PID_Interface2015b/Level Process Recieve Data Protocol/Subsystem Reference8 ==
  LSB : Inport  OutDataTypeStr=uint8
  MSB : Inport  Port=2  OutDataTypeStr=uint8
  Add : Sum
  Data Type Conversion : DataTypeConversion  OutDataTypeStr=uint16
  Data Type Conversion1 : DataTypeConversion  OutDataTypeStr=uint16
  Display{,1..4} (5 alike) : Display
  Shift Arithmetic : ArithShift  BitShiftNumber=8  BitShiftDirection=Left
  UINT16 : Outport  OutDataTypeStr=uint16  LockScale=on
  wires:
  LSB/1 -> Data Type Conversion/1, Display/1
  Shift Arithmetic/1 -> Add/2, Display3/1
  Data Type Conversion/1 -> Add/1, Display2/1
  Add/1 -> UINT16/1, Display4/1
  MSB/1 -> Data Type Conversion1/1, Display1/1
  Data Type Conversion1/1 -> Shift Arithmetic/1

== system Arduino_PID_Interface2015b/Level Process Recieve Data Protocol/Subsystem Reference9 ==
  LSB : Inport  OutDataTypeStr=uint8
  MSB : Inport  Port=2  OutDataTypeStr=uint8
  Add : Sum
  Data Type Conversion : DataTypeConversion  OutDataTypeStr=uint16
  Data Type Conversion1 : DataTypeConversion  OutDataTypeStr=uint16
  Display{,1..4} (5 alike) : Display
  Shift Arithmetic : ArithShift  BitShiftNumber=8  BitShiftDirection=Left
  UINT16 : Outport  OutDataTypeStr=uint16  LockScale=on
  wires:
  LSB/1 -> Data Type Conversion/1, Display/1
  Shift Arithmetic/1 -> Add/2, Display3/1
  Data Type Conversion/1 -> Add/1, Display2/1
  Add/1 -> UINT16/1, Display4/1
  MSB/1 -> Data Type Conversion1/1, Display1/1
  Data Type Conversion1/1 -> Shift Arithmetic/1

== system Arduino_PID_Interface2015b/Level Process Recieve Data Protocol/Subsystem Reference1/Subsystem Reference ==
  LSB : Inport  OutDataTypeStr=uint8
  MSB : Inport  Port=2  OutDataTypeStr=uint8
  Add : Sum
  Data Type Conversion : DataTypeConversion  OutDataTypeStr=uint16
  Data Type Conversion1 : DataTypeConversion  OutDataTypeStr=uint16
  Display{,1..4} (5 alike) : Display
  Shift Arithmetic : ArithShift  BitShiftNumber=8  BitShiftDirection=Left
  UINT16 : Outport  OutDataTypeStr=uint16  LockScale=on
  wires:
  Data Type Conversion1/1 -> Shift Arithmetic/1
  MSB/1 -> Display1/1, Data Type Conversion1/1
  Add/1 -> Display4/1, UINT16/1
  Data Type Conversion/1 -> Display2/1, Add/1
  Shift Arithmetic/1 -> Display3/1, Add/2
  LSB/1 -> Display/1, Data Type Conversion/1

== system Arduino_PID_Interface2015b/Level Process Recieve Data Protocol/Subsystem Reference1/Subsystem Reference1 ==
  LSB : Inport  OutDataTypeStr=uint8
  MSB : Inport  Port=2  OutDataTypeStr=uint8
  Add : Sum
  Data Type Conversion : DataTypeConversion  OutDataTypeStr=uint16
  Data Type Conversion1 : DataTypeConversion  OutDataTypeStr=uint16
  Display{,1..4} (5 alike) : Display
  Shift Arithmetic : ArithShift  BitShiftNumber=8  BitShiftDirection=Left
  UINT16 : Outport  OutDataTypeStr=uint16  LockScale=on
  wires:
  Data Type Conversion1/1 -> Shift Arithmetic/1
  MSB/1 -> Display1/1, Data Type Conversion1/1
  Add/1 -> Display4/1, UINT16/1
  Data Type Conversion/1 -> Display2/1, Add/1
  Shift Arithmetic/1 -> Display3/1, Add/2
  LSB/1 -> Display/1, Data Type Conversion/1

== matlab function Arduino_PID_Interface2015b/Comments To The Setup ==
  data: u input; y output
% DHBW Mosbach
% Mechatronische Systeme 4
% Dr.-Ing. Vanessa Romero Segovia
% MT17B Gruppe 3 (Sarah Plieninger, Fabian Redaoui, Raphael Kuttruf)

function y = fcn(u)

% Actuator overwrite can be used to measure the Step Response

% Gamma is only applied if the Filter is on Bypass

% If Time Sync is connected a CntrolSample is send 
% every Time an new DataSample arrives
% If A Zero Order Hold block is needed 
% in front of the Serial Send Block if you want to send 
% a Control Sample every X-times a DataSample arrives

%  Dont use the INT De-/Serialize Blocks ! They don't work correctly 
% Serializing signed and unsigned integers at the same time is not so easy

y = u;
